simulink model "ProposedProblem7"  (R2013a)
settings: Solver=ode45  StartTime=0.0  StopTime=100.0  RelTol=1e-3
settings Model: Creator=gabig  LastModifiedBy=gabig

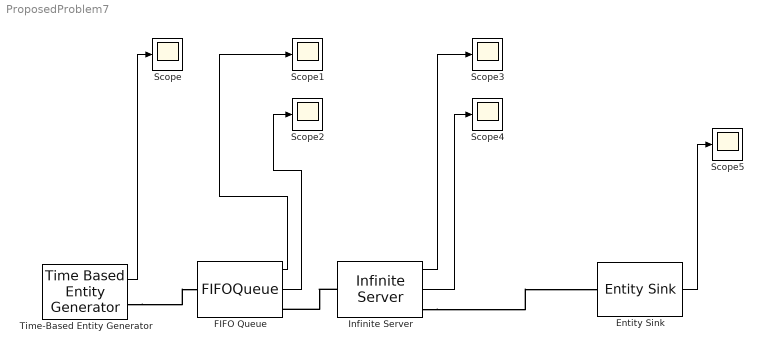
== system ProposedProblem7 ==
  Entity Sink : EntitySink  StatNumberArrived=on
  FIFO Queue : FIFOQueue  StatNumberDeparted=on  StatNumberInBlock=on
      settings: OutputPortMap=o0,o1
  Infinite Server : InfiniteServer  StatNumberDeparted=on  StatNumberInBlock=on
      settings: OutputPortMap=o0,o1
  Scope{,1..5} (6 alike) : Scope
      Scope2 settings: SaveName=ScopeData2
      Scope3 settings: SaveName=ScopeData3
      Scope4 settings: SaveName=ScopeData4
      Scope5 settings: SaveName=ScopeData5
  Time-Based Entity Generator : TimeBasedEntityGenerator  Distribution=Exponential  Mean=0.2  StatNumberDeparted=on
  wires:
  Time-Based Entity Generator/1 -> Scope/1
  FIFO Queue/1 -> Scope1/1
  FIFO Queue/2 -> Scope2/1
  Infinite Server/1 -> Scope3/1
  Infinite Server/2 -> Scope4/1
  Entity Sink/1 -> Scope5/1
  connections:
  Time-Based Entity Generator/RConn1 -- FIFO Queue/LConn1
  Infinite Server/LConn1 -- FIFO Queue/RConn1
  Infinite Server/RConn1 -- Entity Sink/LConn1
